simulink model "lateral_teste"  (R2023a)
settings: Solver=ode4  StartTime=0.0  StopTime=50  FixedStep=0.05  RelTol=1e-3
InitFcn:
  | load('data/refPath.mat')
undefined symbols (not defined in the file): curvature, direction, distancia_eixo_ftraseiro_centro_massa, gradbp, massa, numero_de_eixos_frente, numero_de_eixos_traseira, psi_o, thetaRefs, velt_res, X_o, xRef2s, Y_o, yRef2s
libraries: simulink_extras x3, simulink x2, vehdynlibviscommon x1, checkpacklib x1, drivingvehiclecontroller x1, autolibshared x1
settings Model: DataDictionary=modelo_bike_r23a.sldd  Creator=thailon  LastModifiedBy=thailon

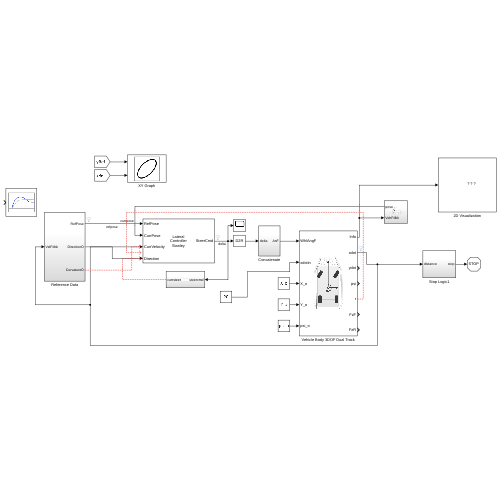
[thumbnail: Simulink's stored preview of the top-level diagram]
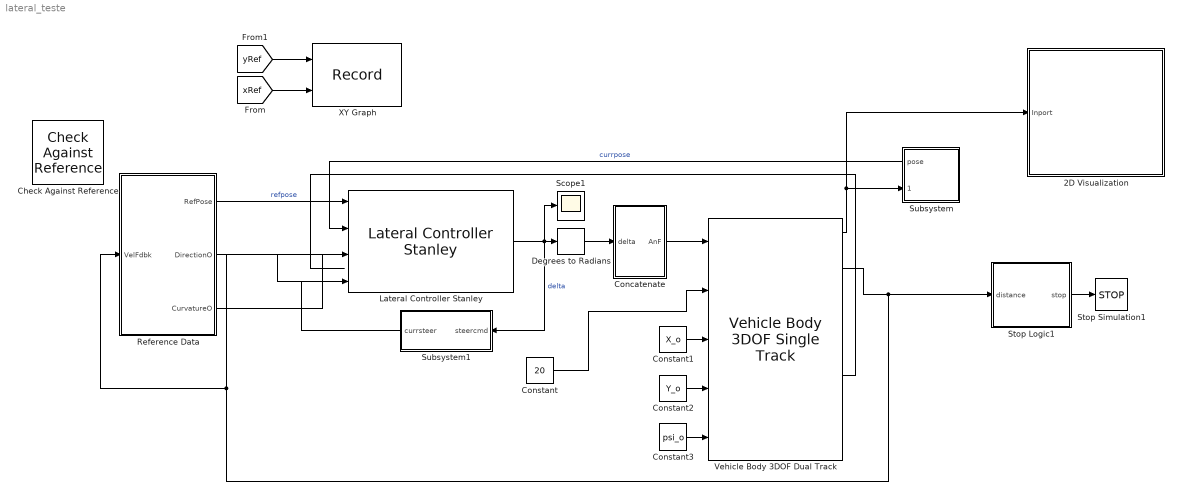
== system lateral_teste ==
  2D Visualization : Subsystem
      mask Display: image("visualization.JPG");
  Check Against Reference : checkpacklib/Check Against Reference  InstantiateOnLoad=on  enabled=on  stopWhenAssertionFail=off  export=off  ViewDlgPos=[]  OpenViewOnLoad=off  LaunchViewOnOpen=off  TimeUnits=seconds  EnableReferenceBound=on  AbsTolerance=eps^(1/3)  RelTolerance=0.01  ReferenceTimes=linspace(0,10)  ReferenceAmplitudes=1-exp(-linspace(0,10)/2)
      settings: LibrarySourceBlock=sdolib/Model Verification/Check Against Reference
  Concatenate : Subsystem
  Constant : Constant  Value=20
  Constant1 : Constant  Value=X_o
  Constant2 : Constant  Value=Y_o
  Constant3 : Constant  Value=psi_o
  Degrees to Radians : simulink_extras/Transformations/Degrees to Radians
  Lateral Controller Stanley : drivingvehiclecontroller/Lateral Controller Stanley  ModelType=Dynamic bicycle model  PositionGainF=stanley_kpfw  PositionGainR=1  YawRateGain=ganho_yaw_rate  DelayGain=ganho_steering  VehicleMass=massa  Lf=distancia_eixo_frontal_centro_massa  Lr=distancia_eixo_ftraseiro_centro_massa  TireStiffness=rigidez_lateral_pneu_frontal  Wheelbase=wheelbase  MaxSteeringAngle=max_steering_angle
  Reference Data : Subsystem  VariantControl=Stanley
  Scope1 : Scope
  Stop Logic1 : Subsystem
  Stop Simulation1 : Stop
  Subsystem : Subsystem
      settings: PortSchema="{\"entries\":[{\"content\":{\"sides\":[{\"content\":{\"connectorIds\":[\"Out1\",\"In1\"]},\"type\":\"ConnectorPlacement.EquallySpacedRectSide\",\"uuid\":\"b99b5404-081b-413b-8715-691cf6906cbd\"},{\"content\":{\"side\":\"RIGHT\"},\"type\":\"ConnectorPlacement.EquallySpacedRectSide\",\"uuid\":\"44ae264f-bc35-4d6a-b735-b6c150e7b378\"},{\"content\":{\"side\":\"TOP\"},\"type\":\"ConnectorPlacement.EquallySpacedRectSide\",\"uuid\":\"02beee6b-e892-461e-bd21-f2bfa96f1776\"}]},\"type\":\"ConnectorPlacement.EquallySpacedConnector\",\"uuid\":\"e0ea02da-d749-438f-a103-031e8afedff8\"}],\"packageUris\":[\"http://schema.mathworks.com/mf0/Connector/R2020b\"],\"version\":\"1.0\"}"
  Subsystem1 : Subsystem
  Vehicle Body 3DOF Dual Track : autolibshared/Vehicle Body 3DOF Single Track  trackMode=Dual  inputMode=External longitudinal velocity  frontSteerMode=on  rearSteerMode=off  windMode=off  muMode=off  extFMode=off  extMMode=off  htchFMode=off  htchMMode=off  extXo=on  extpsio=on  extxdoto=off  extro=off  extYo=on  extTamb=off  extydoto=off  aMode=2  NF=numero_de_eixos_frente  NR=numero_de_eixos_traseira  m=massa  a=distancia_eixo_frontal_centro_massa  b=distancia_eixo_ftraseiro_centro_massa  h=distancia_chao_plano_centro_massa  dh=1  hh=0.2  X_o=0  xdot_o=velt_res(1)  CalphaMode=on  sigmaMode=on  d=distancia_lateral_linha_gemetrica_centro_massa  hl=0  w=bitola  Cy_f=rigidez_lateral_pneu_frontal  Cy_r=rigidez_lateral_pneu_traseira  sigma_f=comprimento_relaxacao_frontal  sigma_r=comprimento_relaxacao_traseira  alpha_f_brk=[-.1 .1]  Cy_f_data=[-9e3 9e3]  alpha_r_brk=[-.1 .1]  Cy_r_data=[-9e3 9e3]  Y_o=0  ydot_o=0  Izz=inercial_polar_yaw  psi_o=0  r_o=giro_yaw_inicial  Af=area_arrasto_longitudinal  Cd=coeficiente_longitudinal_arrasto  Cl=coefficient_longitudinal_sustentacao  Cpm=arrasto_longitudinal_pitch  beta_w=[0:0.01:0.3]  Cs=[0:0.03:0.9]  Cym=[0:0.01:0.3]  Pabs=101325  Tair=273  g=9.81  mu=1  xdot_tol=.01  Fznom=5000  Fxtire_sat=7e4  Fytire_sat=7e4  longOff=0  latOff=0  vertOff=0  wrapAng=off
  XY Graph : Record  FileSettingsInternal="{\"entries\":[{\"content\":{\"excelSettings\":{\"content\":{},\"type\":\"Streamout.ExcelSettings\"}},\"type\":\"Streamout.FileSettingStorage\",\"uuid\":\"\"}],\"packageUris\":[\"http:\\/\\/schema.mathworks.com\\/mf0\\/streamout_blocks\\/R2020a\"],\"version\":\"1.0\"}"  Layout=[1 1]  SignalsInternal="{\"entries\":[{\"content\":{\"signals\":[{\"content\":{\"blockPath\":[],\"dimensions\":[1],\"domain\":\"\",\"lineColor\":\"#a2142f\",\"plots\":[1],\"port\":1,\"signalID\":8,\"signalName\":\"From1\"},\"type\":\"RecordBlkView.Signal\",\"uuid\":\"\"},{\"content\":{\"blockPath\":[],\"dimensions\":[1],\"domain\":\"\",\"lineColor\":\"#139fff\",\"plots\":[1],\"port\":2,\"signalID\":11,\"signalName\":\"From\"},\"type\":\"RecordBlkView.Signal\",\"uuid\":\"\"}]},\"type\":\"RecordBlkView.InputSignals\",\"uuid\":\"\"}],\"packageUris\":[\"http:\\/\\/schema.mathworks.com\\/mf0\\/streamout_blocks\\/R2020a\"],\"version\":\"1.0\"}"  VisualizationBindings="{\"xyplotplugin\":{\"info\":[{\"series\":[{\"bindingParametersList\":[{\"parameter\":\"X-Axis\",\"signalID\":8,\"signalName\":\"From1\"},{\"parameter\":\"Y-Axis\",\"signalID\":11,\"signalName\":\"From\"}],\"seriesID\":2702}],\"subplotID\":1}]}}"  CompatibilityTag=XY
  wires:
  Subsystem/1(pose) -> Lateral Controller Stanley/2  "currpose"
  Constant1/1 -> Vehicle Body 3DOF Dual Track/3
  Reference Data/1(RefPose) -> Lateral Controller Stanley/1  "refpose"
  Vehicle Body 3DOF Dual Track/2 -> Stop Logic1/1(distance), Reference Data/1(VelFdbk), Lateral Controller Stanley/3
  Concatenate/1(AnF) -> Vehicle Body 3DOF Dual Track/1
  Stop Logic1/1(stop) -> Stop Simulation1/1
  Constant3/1 -> Vehicle Body 3DOF Dual Track/5
  Reference Data/2(DirectionO) -> Lateral Controller Stanley/4
  Vehicle Body 3DOF Dual Track/1 -> 2D Visualization/1(Inport), Subsystem/1(VehFdbk)
  Lateral Controller Stanley/1 -> Degrees to Radians/1, Scope1/1, Subsystem1/1(steercmd)  "delta"
  Constant2/1 -> Vehicle Body 3DOF Dual Track/4
  Degrees to Radians/1 -> Concatenate/1(delta)
  Constant/1 -> Vehicle Body 3DOF Dual Track/2
  Reference Data/3(CurvatureO) -> ?
  Vehicle Body 3DOF Dual Track/5 -> ?
  Subsystem1/1(currsteer) -> ?
  [xRef] -> XY Graph/2
  [yRef] -> XY Graph/1

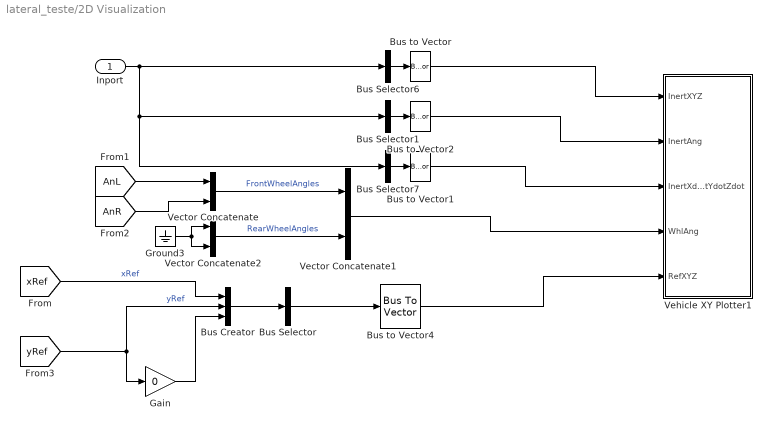
== system lateral_teste/2D Visualization ==
  Inport : Inport
  Bus Creator : BusCreator  Inputs=3
  Bus Selector : BusSelector  OutputSignals=xRef,yRef,signal3  OutputAsBus=on
  Bus Selector1 : BusSelector  OutputSignals=InertFrm.Cg.Ang.phi,InertFrm.Cg.Ang.theta,InertFrm.Cg.Ang.psi  OutputAsBus=on
  Bus Selector6 : BusSelector  OutputSignals=InertFrm.Geom.Disp.X,InertFrm.Geom.Disp.Y,InertFrm.Geom.Disp.Z  OutputAsBus=on
  Bus Selector7 : BusSelector  OutputSignals=InertFrm.Geom.Vel.Xdot,InertFrm.Geom.Vel.Ydot,InertFrm.Geom.Vel.Zdot  OutputAsBus=on
  Bus to Vector{,1..2,4} (4 alike) : BusToVector
  Gain : Gain  Gain=0
  Ground3 : Ground
  Vector Concatenate : Concatenate
  Vector Concatenate1 : Concatenate
  Vector Concatenate2 : Concatenate
  Vehicle XY Plotter1 : Subsystem  mask(Vehicle XY Plotter){extRef=on, extStats=off, extTireF=off, a=numero_de_eixos_frente, b=numero_de_eixos_traseira, w=1.6, figBorder=5, bufferSize=1024, velNorm=5, tireFNorm=1000, pltDT=0.1}
      mask prompts: extRef "Plot path reference, extRef"; extStats "Display speed, RPM and Gear"; extTireF "Display tire forces"; a "Distance to front axle from CG, a [m]:"; b "Distance to rear axle from CG, b [m]:"; w "Track width, w [m]:"; figBorder "Distance to figure borders, figBorder [m]:"; bufferSize "Path buffer sampe size, bufferSize []:"; velNorm "Velocity vector scaling, velNorm [m*s/m]:"; tireFNorm "Tire force vector scaling, tireFNorm [m/N]:"; pltDT "Plot update rate, pltDT [s]:"
      mask help:
      | This block will display a MATLAB figure which indicates the vehicle path, current position and heading velocity.
      | An optional path reference is also provided.
      mask init:
      | block = gcb;
      | if autoblkschecksimstopped(block)
      |     ParamNames = {'extRef';'extStats';'extTireF';'extTireF'};
      |     PortNames = {'RefXYZ';'Stats';'TireFx';'TireFy'};
      |     for idx=1:length(PortNames)
      |         InportOption  = {'built-in/Ground', [PortNames{idx}, ' Ground'];...
      |             'built-in/Inport',PortNames{idx}};
      |         if ~strcmp(get_param(block,ParamNames{idx}),'on')
      |             NewBlkHdl = autoblksreplaceblock(block, InportOption, 1);
      |             set_param(NewBlkHdl, 'ShowName', 'off');
      |         else
      |             autoblksreplaceblock(block, InportOption, 2);
      |         end
      |     end
      |     InportNames = {'InertXYZ';'InertAng';'InertXdotYdotZdot';'WhlAng';'RefXYZ';'Stats';'TireFx';'TireFy'};
      |     FoundNames = get_param(find_system(block, 'LookUnderMasks', 'all', 'SearchDepth', 1, 'FollowLinks', 'on', 'BlockType', 'Inport'), 'Name');
      |     [~,PortI] = intersect(InportNames, FoundNames);
      |     PortI = sort(PortI);
      |     for idx = 1:length(PortI)
      |         set_param([block, '/', InportNames{PortI(idx)}], 'Port', num2str(idx));
      |     end
      | end
      mask TypeOptions a: Vehicle XY Plotter/a
      mask TypeOptions b: Vehicle XY Plotter/b
      mask TypeOptions w: Vehicle XY Plotter/w
      mask TypeOptions figBorder: Vehicle XY Plotter/figBorder
      mask TypeOptions bufferSize: Vehicle XY Plotter/bufferSize
      mask TypeOptions velNorm: Vehicle XY Plotter/velNorm
      mask TypeOptions tireFNorm: Vehicle XY Plotter/tireFNorm
      mask DialogControl Container3 Prompt: Plot and Display Options
  wires:
  Bus Creator/1 -> Bus Selector/1
  [xRef] -> Bus Creator/1  "xRef"
  Gain/1 -> Bus Creator/3
  [yRef] -> Gain/1, Bus Creator/2  "yRef"
  Bus Selector/1 -> Bus to Vector4/1
  Bus to Vector4/1 -> Vehicle XY Plotter1/5(RefXYZ)
  Inport/1 -> Bus Selector6/1, Bus Selector1/1, Bus Selector7/1
  [AnR] -> Vector Concatenate/2
  Bus Selector1/1 -> Bus to Vector2/1
  Bus to Vector2/1 -> Vehicle XY Plotter1/2(InertAng)
  Bus to Vector/1 -> Vehicle XY Plotter1/1(InertXYZ)
  Bus to Vector1/1 -> Vehicle XY Plotter1/3(InertXdotYdotZdot)
  Bus Selector7/1 -> Bus to Vector1/1
  Vector Concatenate2/1 -> Vector Concatenate1/2  "RearWheelAngles"
  [AnL] -> Vector Concatenate/1
  Vector Concatenate/1 -> Vector Concatenate1/1  "FrontWheelAngles"
  Bus Selector6/1 -> Bus to Vector/1
  Ground3/1 -> Vector Concatenate2/2, Vector Concatenate2/1
  Vector Concatenate1/1 -> Vehicle XY Plotter1/4(WhlAng)

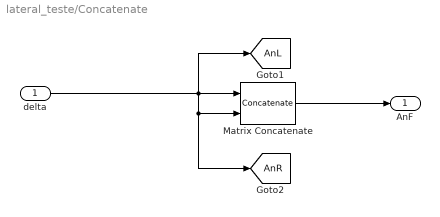
== system lateral_teste/Concatenate ==
  delta : Inport
  Matrix Concatenate : Concatenate
  AnF : Outport  VectorParamsAs1DForOutWhenUnconnected=off
  tag scope: AnL=global, AnR=global
  wires:
  Matrix Concatenate/1 -> AnF/1
  delta/1 -> Matrix Concatenate/1, [AnR], Matrix Concatenate/2, [AnL]

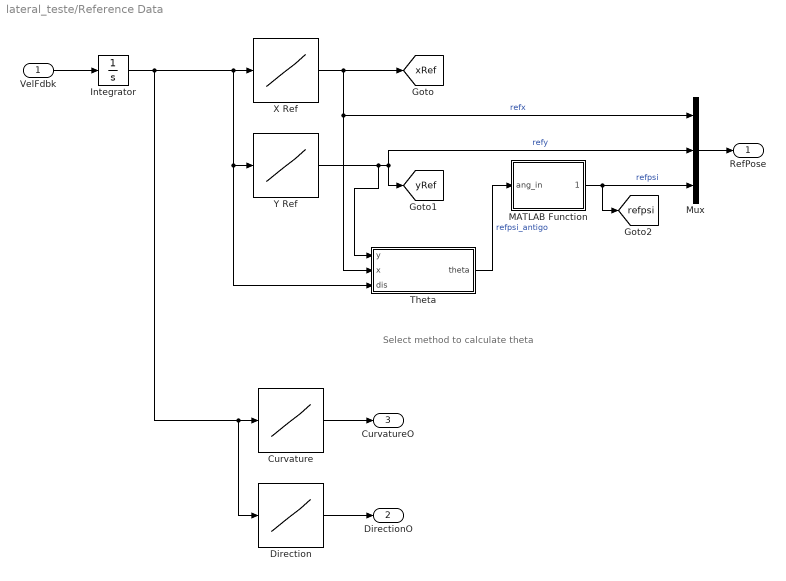
== system lateral_teste/Reference Data ==
  note: Select method to calculate theta
  VelFdbk : Inport
  Curvature : Lookup_n-D  NumberOfTableDimensions=1  BreakpointsForDimension1=gradbp  Table=curvature  InternalRulePriority=Speed  RndMeth=Simplest
  Direction : Lookup_n-D  NumberOfTableDimensions=1  BreakpointsForDimension1=gradbp  Table=direction  InternalRulePriority=Speed  RndMeth=Simplest
  Integrator : Integrator
  MATLAB Function : MATLAB Function  TreatAsAtomicUnit=on
  Mux : Mux  Inputs=3
  Theta : Subsystem  Variant=on  VariantControlMode=label  LabelModeActiveChoice=thetaSimulinkBlock
  X Ref : Lookup_n-D  NumberOfTableDimensions=1  BreakpointsForDimension1=gradbp  Table=xRef2s  ExtrapMethod=Clip  InternalRulePriority=Speed  RndMeth=Simplest
  Y Ref : Lookup_n-D  NumberOfTableDimensions=1  BreakpointsForDimension1=gradbp  Table=yRef2s  InternalRulePriority=Speed  RndMeth=Simplest
  RefPose : Outport
  DirectionO : Outport  Port=2
  CurvatureO : Outport  Port=3
  tag scope: refpsi=global, xRef=global, yRef=global
  wires:
  Direction/1 -> DirectionO/1
  Curvature/1 -> CurvatureO/1
  Y Ref/1 -> Theta/1(y), Mux/2, [yRef]  "refy"
  Mux/1 -> RefPose/1
  X Ref/1 -> Theta/2(x), Mux/1, [xRef]  "refx"
  Integrator/1 -> Curvature/1, Direction/1, Theta/3(dis), Y Ref/1, X Ref/1
  VelFdbk/1 -> Integrator/1
  Theta/1(theta) -> MATLAB Function/1(ang_in)  "refpsi_antigo"
  MATLAB Function/1(ang_out) -> [refpsi], Mux/3  "refpsi"

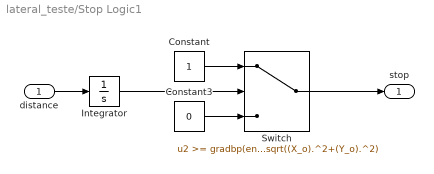
== system lateral_teste/Stop Logic1 ==
  distance : Inport
  Constant : Constant
  Constant3 : Constant  Value=0
  Integrator : Integrator  InitialCondition=sqrt((X_o).^2+(Y_o).^2)
  Switch : Switch  Threshold=gradbp(end)+sqrt((X_o).^2+(Y_o).^2)  SaturateOnIntegerOverflow=off  InputSameDT=off
  stop : Outport
  wires:
  Switch/1 -> stop/1
  Constant3/1 -> Switch/3
  distance/1 -> Integrator/1
  Constant/1 -> Switch/1
  Integrator/1 -> Switch/2

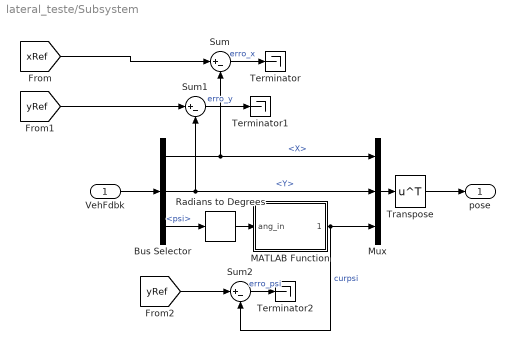
== system lateral_teste/Subsystem ==
  VehFdbk : Inport
  Bus Selector : BusSelector  OutputSignals=InertFrm.Cg.Disp.X,InertFrm.Cg.Disp.Y,InertFrm.Cg.Ang.psi
  MATLAB Function : MATLAB Function  TreatAsAtomicUnit=on
  Mux : Mux  Inputs=3
  Radians to Degrees : simulink_extras/Transformations/Radians to Degrees
  Sum : Sum  Inputs=|+-
  Sum1 : Sum  Inputs=|+-
  Sum2 : Sum  Inputs=|+-
  Terminator : Terminator
  Terminator1 : Terminator
  Terminator2 : Terminator
  Transpose : Math  Operator=transpose  SignedPower=on
  pose : Outport
  wires:
  Mux/1 -> Transpose/1
  VehFdbk/1 -> Bus Selector/1
  Bus Selector/1 -> Sum/2, Mux/1  "<X>"
  Bus Selector/2 -> Sum1/2, Mux/2  "<Y>"
  Transpose/1 -> pose/1
  Bus Selector/3 -> Radians to Degrees/1  "<psi>"
  [xRef] -> Sum/1
  [yRef] -> Sum1/1
  Sum1/1 -> Terminator1/1  "erro_y"
  Sum/1 -> Terminator/1  "erro_x"
  [yRef] -> Sum2/1
  Sum2/1 -> Terminator2/1  "erro_psi"
  Radians to Degrees/1 -> MATLAB Function/1(ang_in)
  MATLAB Function/1(ang_out) -> Mux/3, Sum2/2  "curpsi"

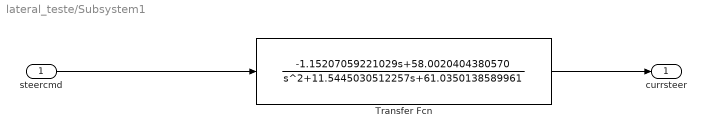
== system lateral_teste/Subsystem1 ==
  steercmd : Inport
  Transfer Fcn : TransferFcn  Numerator="[-1.15207059221029,\t58.0020404380570]"  Denominator="[1,\t11.5445030512257,\t61.0350138589961]"  ParameterTunability=Unconstrained
  currsteer : Outport
  wires:
  steercmd/1 -> Transfer Fcn/1
  Transfer Fcn/1 -> currsteer/1

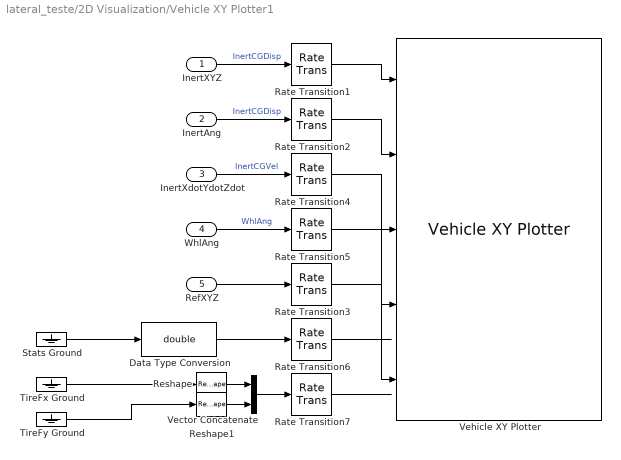
== system lateral_teste/2D Visualization/Vehicle XY Plotter1 ==
  InertXYZ : Inport
  InertAng : Inport  Port=2
  InertXdotYdotZdot : Inport  Port=3
  WhlAng : Inport  Port=4
  RefXYZ : Inport  Port=5
  Data Type Conversion : DataTypeConversion  OutDataTypeStr=double  SaturateOnIntegerOverflow=off  RndMeth=Floor
  Rate Transition{1..7} (7 alike) : RateTransition  Deterministic=off  OutPortSampleTime=pltDT
  Reshape : Reshape  OutputDimensionality=Row vector (2-D)
  Reshape1 : Reshape  OutputDimensionality=Row vector (2-D)
  Stats Ground : Ground
  TireFx Ground : Ground
  TireFy Ground : Ground
  Vector Concatenate : Concatenate  Mode=Multidimensional array
  Vehicle XY Plotter : vehdynlibviscommon/Vehicle XY Plotter  w=w  a=a  b=b  figBorder=figBorder  bufferSize=bufferSize  extStats=off  extTireF=off
  wires:
  InertAng/1 -> Rate Transition2/1  "InertCGDisp"
  InertXdotYdotZdot/1 -> Rate Transition4/1  "InertCGVel"
  InertXYZ/1 -> Rate Transition1/1  "InertCGDisp"
  WhlAng/1 -> Rate Transition5/1  "WhlAng"
  Rate Transition3/1 -> Vehicle XY Plotter/5
  Rate Transition1/1 -> Vehicle XY Plotter/1
  Rate Transition2/1 -> Vehicle XY Plotter/2
  Rate Transition4/1 -> Vehicle XY Plotter/3
  Rate Transition5/1 -> Vehicle XY Plotter/4
  Rate Transition6/1 -> ?
  Data Type Conversion/1 -> Rate Transition6/1
  Rate Transition7/1 -> ?
  RefXYZ/1 -> Rate Transition3/1
  Reshape/1 -> Vector Concatenate/1
  Reshape1/1 -> Vector Concatenate/2
  Vector Concatenate/1 -> Rate Transition7/1
  Stats Ground/1 -> Data Type Conversion/1
  TireFx Ground/1 -> Reshape/1
  TireFy Ground/1 -> Reshape1/1

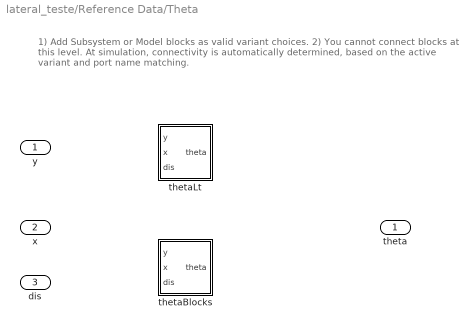
== system lateral_teste/Reference Data/Theta ==
  note: 1) Add Subsystem or Model blocks as valid variant choices.
      | 2) You cannot connect blocks at this level. At simulation, connectivity is automatically
      | determined, based on the active variant and port name matching.
  y : Inport
  x : Inport  Port=2
  dis : Inport  Port=3
  thetaBlocks : Subsystem  VariantControl=thetaSimulinkBlock
  thetaLt : Subsystem  VariantControl=thetaLookUpTable
  theta : Outport

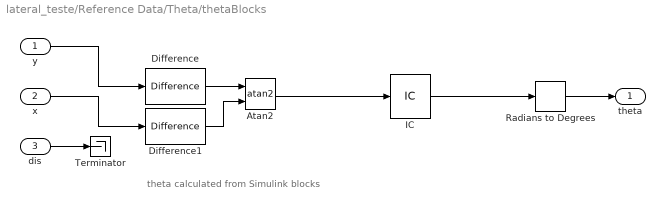
== system lateral_teste/Reference Data/Theta/thetaBlocks ==
  note: theta calculated from Simulink blocks
  y : Inport
  x : Inport  Port=2
  dis : Inport  Port=3
  Atan2 : Trigonometry  Operator=atan2  ApproximationMethod=CORDIC
  Difference : simulink/Discrete/Difference  ICPrevInput=0.0  OutMin=[]  OutMax=[]  OutDataType=fixdt(1, 16)  OutScaling=2^-10  DoSatur=off
  Difference1 : simulink/Discrete/Difference  ICPrevInput=0.0  OutMin=[]  OutMax=[]  OutDataType=fixdt(1, 16)  OutScaling=2^-10  DoSatur=off
  IC : InitialCondition  Value=psi_o
  Radians to Degrees : simulink_extras/Transformations/Radians to Degrees
  Terminator : Terminator
  theta : Outport
  wires:
  IC/1 -> Radians to Degrees/1
  Atan2/1 -> IC/1
  dis/1 -> Terminator/1
  x/1 -> Difference1/1
  y/1 -> Difference/1
  Radians to Degrees/1 -> theta/1
  Difference/1 -> Atan2/1
  Difference1/1 -> Atan2/2

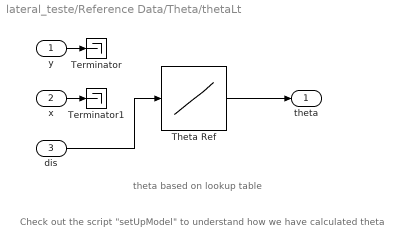
== system lateral_teste/Reference Data/Theta/thetaLt ==
  note: Check out the script "setUpModel" to understand how we have calculated theta
  note: theta based on lookup table
  y : Inport
  x : Inport  Port=2
  dis : Inport  Port=3
  Terminator : Terminator
  Terminator1 : Terminator
  Theta Ref : Lookup_n-D  NumberOfTableDimensions=1  BreakpointsForDimension1=gradbp  Table=thetaRefs  InternalRulePriority=Speed  RndMeth=Simplest
  theta : Outport
  wires:
  Theta Ref/1 -> theta/1
  dis/1 -> Theta Ref/1
  x/1 -> Terminator1/1
  y/1 -> Terminator/1

== matlab function lateral_teste/Reference Data/MATLAB Function ==
  data: ang_in input; ang_out output
function ang_out = fixAngle(ang_in)
    ang_out = mod(ang_in, 360);
    if ang_out < 0
        ang_out = ang_out + 360;
    end
end

== matlab function lateral_teste/Subsystem/MATLAB Function ==
  data: ang_in input; ang_out output
function ang_out = fixAngle(ang_in)
    ang_out = mod(ang_in, 360);
    if ang_out < 0
        ang_out = ang_out + 360;
    end
end
